simulink model "block_diagram_Series"  (R2023b)
settings: Solver=VariableStepAuto  StartTime=0.0  StopTime=2  RelTol=1e-3
values from neighbouring files (symbols this model uses):
  Bm = 0.0025    [setup_params_series.m]
  J = 0.02365    [setup_params_series.m]
  LAA = 0.12    [setup_params_series.m]
  LAF = 0.0675    [setup_params_series.m]
  LFF = 0.03    [setup_params_series.m]
  ra = 1.5    [setup_params_series.m]
  rf = 0.7    [setup_params_series.m]
  Tl = 10    [setup_params_series.m]
  Va = 100    [setup_params_series.m]
  Vf = 100    [setup_params_series.m]
settings Model: Creator=Noor  LastModifiedBy=USER
settings SolverCC: AlgebraicLoopSolver=TrustRegion
settings DataIOCC: ReturnWorkspaceOutputs=off
settings DebuggingCC: UnconnectedInputMsg=warning  UnconnectedOutputMsg=warning  UnconnectedLineMsg=warning  ArithmeticOperatorsInVariantConditions=warning
settings ModelReferenceCC: EnableRefExpFcnMdlSchedulingChecks=on
settings SFSimCC: SimUseLocalCustomCode=off  CustomCodeUndefinedFunction=UseInterfaceOnly
settings RTWCC: RTWUseLocalCustomCode=off

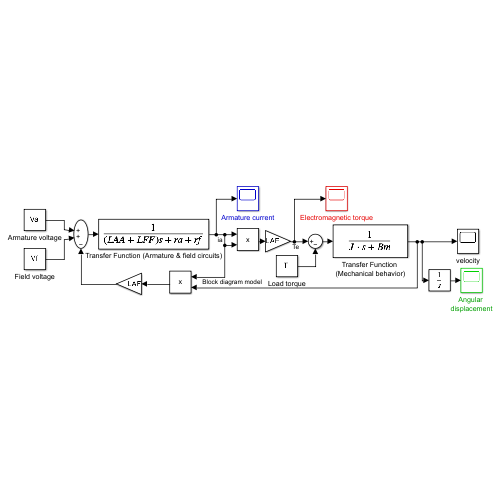
[thumbnail: Simulink's stored preview of the top-level diagram]
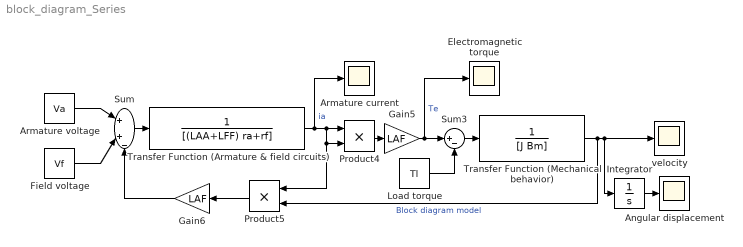
== system block_diagram_Series ==
  Angular displacement : Scope
  Armature current : Scope
  Armature voltage : Constant  Value=Va
  Electromagnetic torque : Scope
  Field voltage : Constant  Value=Vf
  Gain5 : Gain  Gain=LAF
  Gain6 : Gain  Gain=LAF
  Integrator : Integrator
  Load torque : Constant  Value=Tl
  Product4 : Product
  Product5 : Product
  Sum : Sum  Inputs=|++-
  Sum3 : Sum  Inputs=|+-
  Transfer Function (Mechanical behavior) : TransferFcn  Denominator=[J Bm]
  Transfer Function (Armature & field circuits) : TransferFcn  Denominator=[(LAA+LFF) ra+rf]
  velocity : Scope
  wires:
  Transfer Function (Mechanical behavior)/1 -> Product5/2, velocity/1, Integrator/1  "Block diagram model"
  Integrator/1 -> Angular displacement/1
  Gain5/1 -> Electromagnetic torque/1, Sum3/1  "Te"
  Gain6/1 -> Sum/3
  Sum/1 -> Transfer Function (Armature & field circuits)/1
  Armature voltage/1 -> Sum/1
  Transfer Function (Armature & field circuits)/1 -> Armature current/1, Product4/2, Product5/1, Product4/1  "ia"
  Product5/1 -> Gain6/1
  Load torque/1 -> Sum3/2
  Sum3/1 -> Transfer Function (Mechanical behavior)/1
  Product4/1 -> Gain5/1
  Field voltage/1 -> Sum/2
